simulink model "simple_mux_demux"  (Simulink 7.1)
settings: Solver=ode45  StartTime=0.0  StopTime=10.0  RelTol=1e-3
settings Model: Creator=Administrator  LastModifiedBy=Administrator

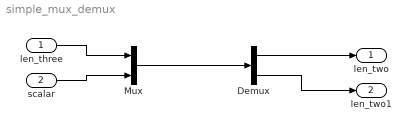
== system simple_mux_demux ==
  len_three : Inport  PortDimensions=[3]  DataType=single  OutDataType=sfix(16)  OutScaling=2^0  OutDataTypeStr=single
  scalar : Inport  Port=2  PortDimensions=[1]  DataType=single  OutDataType=sfix(16)  OutScaling=2^0  OutDataTypeStr=single
  Demux : Demux  Outputs=[2,2]
  Mux : Mux  Inputs=[3,1]
  len_two : Outport  PortDimensions=[2]  DataType=single  OutDataType=sfix(16)  OutScaling=2^0  OutDataTypeStr=single
  len_two1 : Outport  Port=2  PortDimensions=[2]  DataType=single  OutDataType=sfix(16)  OutScaling=2^0  OutDataTypeStr=single
  wires:
  len_three/1 -> Mux/1
  scalar/1 -> Mux/2
  Mux/1 -> Demux/1
  Demux/1 -> len_two/1
  Demux/2 -> len_two1/1
